simulink model "AdaptiveControl"  (Simulink 7.9)
settings: Solver=ode45  StartTime=0.0  StopTime=10.0  RelTol=1e-3
undefined symbols (not defined in the file): DiscIntNeverNeededParam, k1, k2, k3, k4, k5, k6, LinePTs2Rpm, PosSourceSelect, Ts, w1, w2, w3, w4, w5, w6
libraries: powerlib_extras x3
settings Model: Creator=Administrator  LastModifiedBy=Administrator

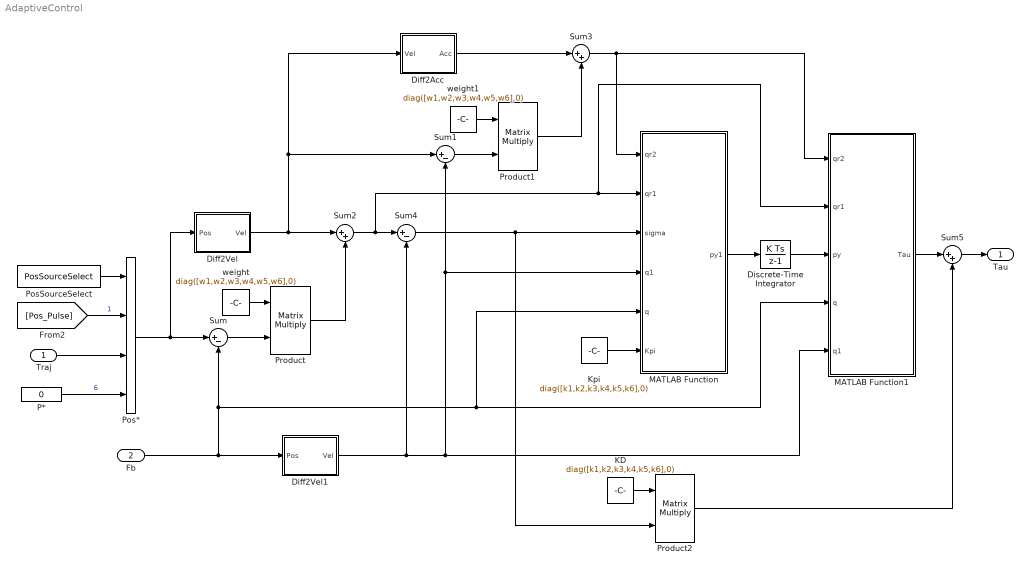
== system AdaptiveControl ==
  Traj : Inport
  Fb : Inport  Port=2
  Diff2Acc : Subsystem
  Diff2Vel : Subsystem
  Diff2Vel1 : Subsystem
  Discrete-Time Integrator : DiscreteIntegrator  ICPrevOutput=DiscIntNeverNeededParam  ICPrevScaledInput=DiscIntNeverNeededParam
  KD : Constant  Value=diag([k1,k2,k3,k4,k5,k6],0)
  Kpi : Constant  Value=diag([k1,k2,k3,k4,k5,k6],0)
  MATLAB Function : MATLAB Function  TreatAsAtomicUnit=on
  MATLAB Function1 : MATLAB Function  TreatAsAtomicUnit=on
  P* : Constant  Value=0  SampleTime=Ts
  Pos* : MultiPortSwitch  zeroidx=off  SampleTime=Ts
  PosSourceSelect : Constant  Value=PosSourceSelect  SampleTime=Ts
  Product : Product  Multiplication=Matrix(*)  RndMeth=Zero
  Product1 : Product  Multiplication=Matrix(*)  RndMeth=Zero
  Product2 : Product  Multiplication=Matrix(*)  RndMeth=Zero
  Sum : Sum  Inputs=|+-  SampleTime=Ts
  Sum1 : Sum  Inputs=|+-  SampleTime=Ts
  Sum2 : Sum  Inputs=|++  SampleTime=Ts
  Sum3 : Sum  Inputs=|++  SampleTime=Ts
  Sum4 : Sum  Inputs=|+-  SampleTime=Ts
  Sum5 : Sum  Inputs=|++  SampleTime=Ts
  weight : Constant  Value=diag([w1,w2,w3,w4,w5,w6],0)
  weight1 : Constant  Value=diag([w1,w2,w3,w4,w5,w6],0)
  Tau : Outport
  wires:
  [Pos_Pulse] -> Pos*/2  "1"
  P*/1 -> Pos*/4  "6"
  PosSourceSelect/1 -> Pos*/1
  Traj/1 -> Pos*/3
  Pos*/1 -> Sum/1, Diff2Vel/1(Pos)
  weight/1 -> Product/1
  Sum/1 -> Product/2
  Product/1 -> Sum2/2
  Diff2Vel/1(Vel) -> Sum2/1, Sum1/1, Diff2Acc/1(Vel)
  weight1/1 -> Product1/1
  Sum1/1 -> Product1/2
  Diff2Acc/1(Acc) -> Sum3/1
  Product1/1 -> Sum3/2
  Fb/1 -> Diff2Vel1/1(Pos), Sum/2, MATLAB Function/5(q), MATLAB Function1/4(q)
  Diff2Vel1/1(Vel) -> Sum4/2, Sum1/2, MATLAB Function/4(q1), MATLAB Function1/5(q1)
  Sum2/1 -> Sum4/1, MATLAB Function/2(qr1), MATLAB Function1/2(qr1)
  Sum4/1 -> MATLAB Function/3(sigma), Product2/2
  Sum3/1 -> MATLAB Function/1(qr2), MATLAB Function1/1(qr2)
  Kpi/1 -> MATLAB Function/6(Kpi)
  MATLAB Function/1(py1) -> Discrete-Time Integrator/1
  Discrete-Time Integrator/1 -> MATLAB Function1/3(py)
  MATLAB Function1/1(Tau) -> Sum5/1
  KD/1 -> Product2/1
  Product2/1 -> Sum5/2
  Sum5/1 -> Tau/1

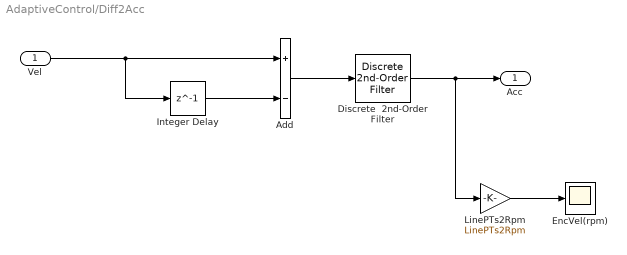
== system AdaptiveControl/Diff2Acc ==
  Vel : Inport
  Add : Sum  Inputs=+-
  Discrete  2nd-Order Filter : powerlib_extras/Discrete  Control Blocks/Discrete  2nd-Order Filter  FilterType=Lowpass  Fo=200  Zeta=0.707  Ts=Ts  Initialize=off  Vac_Init=[0.8 -25 60]  Vdc_Init=-0.4  PlotResponse=off  param1=[1 5000 10]
  EncVel(rpm) : Scope
      settings: SaveName=ScopeData33
  Integer Delay : Delay  DelayLength=1  InputProcessing=Inherited
  LinePTs2Rpm : Gain  Gain=LinePTs2Rpm
  Acc : Outport
  wires:
  Add/1 -> Discrete  2nd-Order Filter/1
  Discrete  2nd-Order Filter/1 -> Acc/1, LinePTs2Rpm/1
  Vel/1 -> Integer Delay/1, Add/1
  Integer Delay/1 -> Add/2
  LinePTs2Rpm/1 -> EncVel(rpm)/1

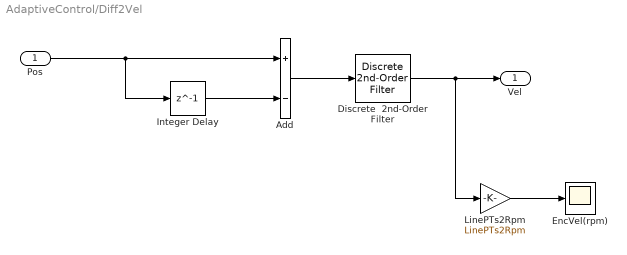
== system AdaptiveControl/Diff2Vel ==
  Pos : Inport
  Add : Sum  Inputs=+-
  Discrete  2nd-Order Filter : powerlib_extras/Discrete  Control Blocks/Discrete  2nd-Order Filter  FilterType=Lowpass  Fo=200  Zeta=0.707  Ts=Ts  Initialize=off  Vac_Init=[0.8 -25 60]  Vdc_Init=-0.4  PlotResponse=off  param1=[1 5000 10]
  EncVel(rpm) : Scope
      settings: SaveName=ScopeData33
  Integer Delay : Delay  DelayLength=1  InputProcessing=Inherited
  LinePTs2Rpm : Gain  Gain=LinePTs2Rpm
  Vel : Outport
  wires:
  Add/1 -> Discrete  2nd-Order Filter/1
  Discrete  2nd-Order Filter/1 -> Vel/1, LinePTs2Rpm/1
  Pos/1 -> Integer Delay/1, Add/1
  Integer Delay/1 -> Add/2
  LinePTs2Rpm/1 -> EncVel(rpm)/1

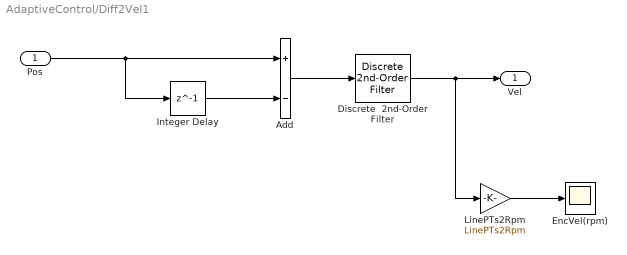
== system AdaptiveControl/Diff2Vel1 ==
  Pos : Inport
  Add : Sum  Inputs=+-
  Discrete  2nd-Order Filter : powerlib_extras/Discrete  Control Blocks/Discrete  2nd-Order Filter  FilterType=Lowpass  Fo=200  Zeta=0.707  Ts=Ts  Initialize=off  Vac_Init=[0.8 -25 60]  Vdc_Init=-0.4  PlotResponse=off  param1=[1 5000 10]
  EncVel(rpm) : Scope
      settings: SaveName=ScopeData33
  Integer Delay : Delay  DelayLength=1  InputProcessing=Inherited
  LinePTs2Rpm : Gain  Gain=LinePTs2Rpm
  Vel : Outport
  wires:
  Add/1 -> Discrete  2nd-Order Filter/1
  Discrete  2nd-Order Filter/1 -> Vel/1, LinePTs2Rpm/1
  Pos/1 -> Integer Delay/1, Add/1
  Integer Delay/1 -> Add/2
  LinePTs2Rpm/1 -> EncVel(rpm)/1

== matlab function MATLAB Function1 ==
  data: qr2 input double; qr1 input double; py input double; q input double; q1 input double; Tau output double
function Tau = fcn(qr2,qr1,py,q,q1)
%#codegen
Tau=Y*py;
end

== matlab function MATLAB Function ==
  data: qr2 input double; qr1 input double; sigma input double; q1 input double; q input double; py1 output double; Kpi input double
function py1 = fcn(qr2,qr1,sigma,q1,q,Kpi)
%#codegen
py1=inv(Kpi)*Y'*sigma;
end
